simulink model "kobuki"  (R2013b)
settings: Solver=VariableStepDiscrete  StartTime=0.0  StopTime=30  MaxStep=1  RelTol=1e-3
settings Model: Creator=lovel  LastModifiedBy=lovel
settings SolverCC: AutoInsertRateTranBlk=on
settings DataIOCC: SaveOutput=off  SaveTime=off
settings OptimizationCC: InlineParams=on  InlineInvariantSignals=on  StateBitsets=on  DataBitsets=on  UseTempVars=on  ZeroExternalMemoryAtStartup=off  ZeroInternalMemoryAtStartup=off  NoFixptDivByZeroProtection=on  OptimizeModelRefInitCode=on  LifeSpan=1
settings HardwareCC: ProdIntDivRoundTo=Floor  ProdEndianess=LittleEndian  ProdHWDeviceType=Generic->Custom
settings RTWCC: SystemTargetFile=ert.tlc  TLCOptions=-p0  GenCodeOnly=on  TemplateMakefile=ert_default_tmf  Description=Embedded Coder  GenerateReport=on  RTWVerbose=off  ProcessScript=ert_make_rtw_hook  IncludeHyperlinkInReport=on  LaunchReport=on
settings CodeAppCC: ForceParamTrailComments=on  IgnoreCustomStorageClasses=off  SimulinkDataObjDesc=on  CustomSymbolStrGlobalVar=rt$N$M  CustomSymbolStrType=$N$M  CustomSymbolStrFcn=$N$M$F  CustomSymbolStrMacro=$N$M  InsertBlockDesc=on
settings ERTTargetCC: CodeReplacementLibrary=ISO_C  GenerateSampleERTMain=on  IncludeMdlTerminateFcn=off  SuppressErrorStatus=on  SupportAbsoluteTime=off  SupportNonFinite=off  SupportComplex=off  PurelyIntegerCode=on  InlinedParameterPlacement=NonHierarchical  RootIOFormat=Structure reference  ERTCustomFileTemplate=example_file_process.tlc

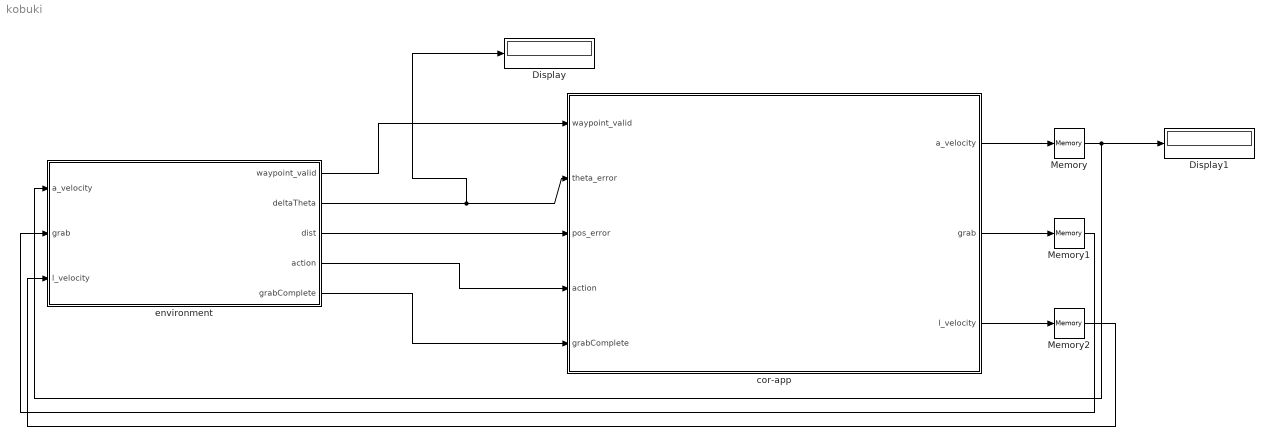
== system kobuki ==
  Display : Display
  Display1 : Display
  Memory : Memory
  Memory1 : Memory
  Memory2 : Memory
  "cor-app " : Stateflow chart  TreatAsAtomicUnit=on
  environment : MATLAB Function  TreatAsAtomicUnit=on
  wires:
  environment/1(waypoint_valid) -> "cor-app "/1(waypoint_valid)
  environment/3(dist) -> "cor-app "/3(pos_error)
  environment/4(action) -> "cor-app "/4(action)
  environment/5(grabComplete) -> "cor-app "/5(grabComplete)
  "cor-app "/1(a_velocity) -> Memory/1
  Memory/1 -> environment/1(a_velocity), Display1/1
  "cor-app "/2(grab) -> Memory1/1
  Memory1/1 -> environment/2(grab)
  "cor-app "/3(l_velocity) -> Memory2/1
  Memory2/1 -> environment/3(l_velocity)
  environment/2(deltaTheta) -> Display/1, "cor-app "/2(theta_error)

== stateflow chart kobuki/cor-app  ==
  note: Inputs:
      | theta_error: R
      | pos_error: R
      | action: enum
      |
      | Variables:
      | timer: R
      |
      | Outputs:
      | a_velocity: R
      | l_velocity: R
      | grab: {0,1}
      | release: {0,1}
  state AlignCW
    during: a_velocity = 1;
  state Stop
    entry:
    l_velocity = 0;
    a_velocity = 0;
    goal_complete = 1;
    exit:
    goal_complete = 0;
  state AlignCCW
    during: a_velocity = -1;
  state Drive
    during: l_velocity = 1;
  state Grab
    entry: timer = 0;
    during: grab = 1;
    timer = timer + 1;
  state Release
    entry: timer = 0
    during: release = 1;
    timer = timer + 1;
  Stop -> Stop [order 2] : [action==3]
  Drive -> AlignCW [order 3]
  Stop -> AlignCW [order 4] : [action==0 && theta_error < 0]
  AlignCW -> Drive : [theta_error <= abs(0.5)]
  Stop -> AlignCCW [order 1] : [action==0 && theta_error > 0]
  (default) -> Stop
  Drive -> Stop [order 2] : [pos_error <= 0.1]
  Stop -> Release [order 5] : [action==2]
  Release -> Stop : [timer >= 5]
  Stop -> Grab [order 3] : [action==1]
  Grab -> Stop : [timer >= 5]
  Drive -> AlignCCW [order 1] : [theta_error >= 0.5]
  AlignCCW -> Drive : [theta_error <= 0.5]
  data: waypoint_valid input; theta_error input double; pos_error input double; grabTime local double; action input; grabComplete input; a_velocity output double; grab output double; l_velocity output double

== matlab function kobuki/environment ==
  data: waypoint_valid output; deltaTheta output; dist output; action output; grabComplete output; a_velocity input; grab input; l_velocity input
function [waypoint_valid, deltaTheta, dist, action, grabComplete] = fcn(a_velocity, grab, l_velocity)
%#codegen

waypoints = [[0,1], [0,2], [3,0]];
curr_waypoint = waypoints(1);

persistent p_deltaTheta
persistent p_dist
if isempty(p_deltaTheta)
    p_deltaTheta = 2;
    p_dist = 3;
end
action = 1; % move
waypoint_valid = 1;


if(grab) 
    grabComplete = 1;
else
    grabComplete = 0;
end

if(a_velocity > 0)
    p_deltaTheta = p_deltaTheta - 1;
end
deltaTheta = p_deltaTheta;

if(l_velocity > 0)
    p_dist = p_dist - 1;
end
dist = p_dist;
